simulink model "sldemo_bpcheck"  (R2024a)
settings: Solver=ode45  StartTime=0.0  StopTime=10.0  RelTol=1e-3  EnableMultiTasking=on
undefined symbols (not defined in the file): membrane
settings Model: Creator=The MathWorks, Inc.  LastModifiedBy=uditpant
settings SolverCC: AlgebraicLoopSolver=TrustRegion
settings DataIOCC: LimitDataPoints=on  SaveFormat=Array  SignalLoggingName=sigsOut
settings OptimizationCC: BooleanDataType=off  ExpressionDepthLimit=2147483647  InitFltsAndDblsToZero=on  LifeSpan=inf
settings DebuggingCC: SaveWithParameterizedLinksMsg=none  CheckExecutionContextPreStartOutputMsg=on  SignalResolutionControl=TryResolveAllWithWarning  MultiTaskDSMMsg=warning  MultiTaskCondExecSysMsg=none  FcnCallInpInsideContextMsg=warning  UnconnectedInputMsg=warning  UnconnectedOutputMsg=warning  UnconnectedLineMsg=warning  StateNameClashWarn=warning  SFUnexpectedBacktrackingDiag=warning  SFNoUnconditionalDefaultTransitionDiag=warning  SFExecutionAtInitializationDiag=none  ArithmeticOperatorsInVariantConditions=warning
settings HardwareCC: ProdBitPerPointer=32  ProdBitPerSizeT=32  ProdBitPerPtrDiffT=32  ProdLargestAtomicFloat=None  ProdIntDivRoundTo=Undefined  ProdEndianess=Unspecified  ProdWordSize=32  ProdHWDeviceType=32-bit Generic  TargetUnknown=on
settings ModelReferenceCC: EnableRefExpFcnMdlSchedulingChecks=on  PropagateSignalLabelsOutOfModel=off
settings SFSimCC: SimUseLocalCustomCode=off  CustomCodeUndefinedFunction=UseInterfaceOnly
settings RTWCC: RTWUseLocalCustomCode=off  GPUComputeCapability=3.5  DLArmComputeVersion=19.05
settings CodeAppCC: StateflowObjectComments=on
settings GRTTargetCC: TargetFcnLib=ansi_tfl_tmw.mat  TargetLangStandard=C89/C90 (ANSI)  CombineOutputUpdateFcns=off  GRTInterface=on
settings ConfigComp: CovMetricSettings=dw  CovSaveCumulativeToWorkspaceVar=on  CovSaveSingleToWorkspaceVar=on  CovExternalEMLEnable=off  CovSFcnEnable=off

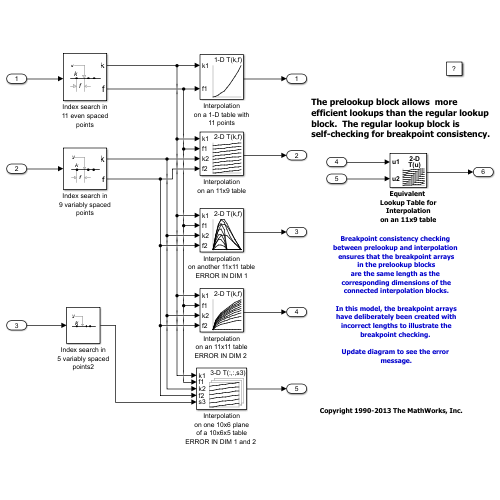
[thumbnail: Simulink's stored preview of the top-level diagram]
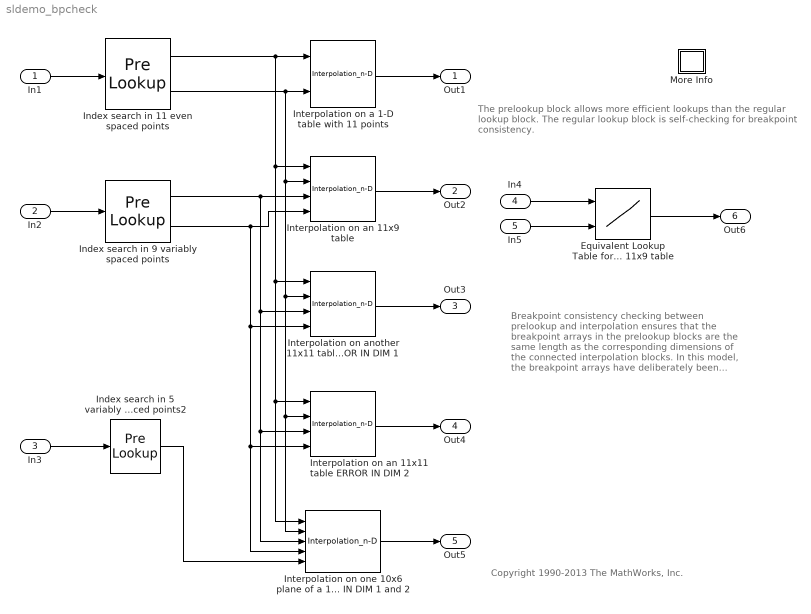
== system sldemo_bpcheck ==
  note: Breakpoint consistency checking
      | between prelookup and interpolation
      | ensures that the breakpoint arrays
      | in the prelookup blocks
      | are the same length as the
      | corresponding dimensions of the
      | connected interpolation blocks.
      |
      | In this model, the breakpoint arrays
      | have deliberately been created with
      |  incorrect lengths to illustrate the
      | breakpoint checking.
      |
      | Update diagram to see the error
      | message.
  note: The prelookup block allows more
      | efficient lookups than the regular lookup
      | block. The regular lookup block is
      | self-checking for breakpoint consistency.
  note: Copyright 1990-2013 The MathWorks, Inc.
  In1 : Inport
  In2 : Inport  Port=2
  In3 : Inport  Port=3
  In4 : Inport  Port=4
  In5 : Inport  Port=5
  Equivalent Lookup Table for Interpolation on an 11x9 table : Lookup_n-D  BreakpointsForDimension1=[0:10:100]  BreakpointsForDimension2=[ 0.5, 1, 3, 5, 15, 45, 95, 96, 97 ]  Table=reshape([1:99], [11,9])  RndMeth=Simplest
      settings: InputPortMap=u0,u1
  Index search in 11 even spaced points : PreLookup  BreakpointsData=[0:10:100]  IndexSearchMethod=Evenly spaced points  ExtrapMethod=Linear
  Index search in 5 variably spaced points2 : PreLookup  BreakpointsData=[-100, 125, 150, 200, 500]  OutputSelection=Index only  IndexSearchMethod=Linear search  BeginIndexSearchUsingPreviousIndexResult=on  DiagnosticForOutOfRangeInput=Warning
  Index search in 9 variably spaced points : PreLookup  BreakpointsData=[ 0.5, 1, 3, 5, 15, 45, 95, 96, 97 ]  BeginIndexSearchUsingPreviousIndexResult=on  ExtrapMethod=Linear
  Interpolation on a 1-D table with 11 points : Interpolation_n-D  NumberOfTableDimensions=1  Table=[1:11].*[1:11]  ExtrapMethod=Clip
      settings: InputPortMap=u0,u1
  "Interpolation on an 11x11 table ERROR IN DIM 2 " : Interpolation_n-D  Table=sqrt([0:10]'*[0:10])
  Interpolation on an 11x9 table : Interpolation_n-D  Table=reshape([1:99], [11,9])  ExtrapMethod=Clip
  Interpolation on another 11x11 table ERROR IN DIM 1 : Interpolation_n-D  Table=membrane(1,5,9,9)
  "Interpolation on one 10x6 plane of a 10x6x5 table ERROR IN DIM 1 and 2 " : Interpolation_n-D  NumberOfTableDimensions=3  Table=reshape([1:300], [10,6,5])  ExtrapMethod=Clip  NumSelectionDims=1
      settings: InputPortMap=u0,u1,u2,u3,u4
  More Info : Subsystem
      settings: OpenFcn=showExample('simulink_features/UsingThePrelookupAndInterpolationBlocksExample')
      mask Display: disp('?')
  Out1 : Outport  VectorParamsAs1DForOutWhenUnconnected=off
  Out2 : Outport  Port=2  VectorParamsAs1DForOutWhenUnconnected=off
  Out3 : Outport  Port=3  VectorParamsAs1DForOutWhenUnconnected=off
  Out4 : Outport  Port=4  VectorParamsAs1DForOutWhenUnconnected=off
  Out5 : Outport  Port=5  VectorParamsAs1DForOutWhenUnconnected=off
  Out6 : Outport  Port=6  VectorParamsAs1DForOutWhenUnconnected=off
  wires:
  In1/1 -> Index search in 11 even spaced points/1
  In2/1 -> Index search in 9 variably spaced points/1
  In3/1 -> Index search in 5 variably spaced points2/1
  Index search in 5 variably spaced points2/1 -> "Interpolation on one 10x6 plane of a 10x6x5 table ERROR IN DIM 1 and 2 "/5
  Interpolation on an 11x9 table/1 -> Out2/1
  Interpolation on another 11x11 table ERROR IN DIM 1/1 -> Out3/1
  "Interpolation on one 10x6 plane of a 10x6x5 table ERROR IN DIM 1 and 2 "/1 -> Out5/1
  Interpolation on a 1-D table with 11 points/1 -> Out1/1
  "Interpolation on an 11x11 table ERROR IN DIM 2 "/1 -> Out4/1
  In4/1 -> Equivalent Lookup Table for Interpolation on an 11x9 table/1
  In5/1 -> Equivalent Lookup Table for Interpolation on an 11x9 table/2
  Equivalent Lookup Table for Interpolation on an 11x9 table/1 -> Out6/1
  Index search in 11 even spaced points/1 -> "Interpolation on one 10x6 plane of a 10x6x5 table ERROR IN DIM 1 and 2 "/1, "Interpolation on an 11x11 table ERROR IN DIM 2 "/1, Interpolation on another 11x11 table ERROR IN DIM 1/1, Interpolation on an 11x9 table/1, Interpolation on a 1-D table with 11 points/1
  Index search in 9 variably spaced points/1 -> "Interpolation on one 10x6 plane of a 10x6x5 table ERROR IN DIM 1 and 2 "/3, "Interpolation on an 11x11 table ERROR IN DIM 2 "/3, Interpolation on another 11x11 table ERROR IN DIM 1/3, Interpolation on an 11x9 table/3
  Index search in 9 variably spaced points/2 -> "Interpolation on one 10x6 plane of a 10x6x5 table ERROR IN DIM 1 and 2 "/4, "Interpolation on an 11x11 table ERROR IN DIM 2 "/4, Interpolation on another 11x11 table ERROR IN DIM 1/4, Interpolation on an 11x9 table/4
  Index search in 11 even spaced points/2 -> "Interpolation on one 10x6 plane of a 10x6x5 table ERROR IN DIM 1 and 2 "/2, "Interpolation on an 11x11 table ERROR IN DIM 2 "/2, Interpolation on another 11x11 table ERROR IN DIM 1/2, Interpolation on an 11x9 table/2, Interpolation on a 1-D table with 11 points/2

== system sldemo_bpcheck/More Info ==
